simulink model "singletrack_ROS"  (R2017b)
settings: Solver=ode2  StartTime=0.0  StopTime=100  FixedStep=ROS_nodePeriod  MaxStep=1e-3  RelTol=1e-4  AbsTol=1e-4
values from neighbouring files (symbols this model uses):
  initial_conditions = [0,0,0,0,0]    [initParameters.m]
  ROS_clockPublishingPeriod = 1.0e-2    (= 0.01)    [initParameters.m]    (also in init_singletrack.m = 0.0005)
  ROS_nodePeriod = 1.0e-3    (= 0.001)    [initParameters.m]
  ROS_statePublishingPeriod = 2.0e-2    (= 0.02)    [initParameters.m]    (also in init_singletrack.m = 0.01)
undefined symbols (not defined in the file or in its folder): Clock_, Theta, X, Y
libraries: robotlib x12, simulink x1
settings Model: ExtModeTrigDuration=100  Creator=Alessandro  LastModifiedBy=bascetta
settings SolverCC: MaxConsecutiveMinStep=10  ZeroCrossControl=DisableAll
settings DataIOCC: SaveFormat=Array  SaveOutput=off  SaveTime=off  StateSaveName=tmp_raccel_xout  TimeSaveName=t_out  SignalLoggingName=SDO_logsout
settings OptimizationCC: EfficientMapNaN2IntZero=off  LifeSpan=inf
settings DebuggingCC: SFUnexpectedBacktrackingDiag=warning  SFNoUnconditionalDefaultTransitionDiag=warning  SFExecutionAtInitializationDiag=none
settings HardwareCC: ProdBitPerPointer=32  ProdBitPerSizeT=32  ProdBitPerPtrDiffT=32  ProdLargestAtomicFloat=None  ProdIntDivRoundTo=Undefined  ProdEndianess=Unspecified  ProdWordSize=32  ProdHWDeviceType=32-bit Generic  TargetBitPerLong=64  TargetBitPerPointer=64  TargetBitPerSizeT=64  TargetBitPerPtrDiffT=64  TargetLongLongMode=on  TargetIntDivRoundTo=Zero  TargetEndianess=LittleEndian  TargetWordSize=64  TargetHWDeviceType=MATLAB Host  ProdEqTarget=off
settings ModelReferenceCC: PropagateSignalLabelsOutOfModel=off
settings CodeAppCC: MaxIdLength=128  StateflowObjectComments=on
settings GRTTargetCC: TargetLangStandard=C89/C90 (ANSI)  GeneratePreprocessorConditionals=Disable all  CombineOutputUpdateFcns=off  GRTInterface=on
settings ConfigComp: CovMetricSettings=dw  CovHtmlReporting=on  CovSaveCumulativeToWorkspaceVar=on  CovSaveSingleToWorkspaceVar=on  CovExternalEMLEnable=off

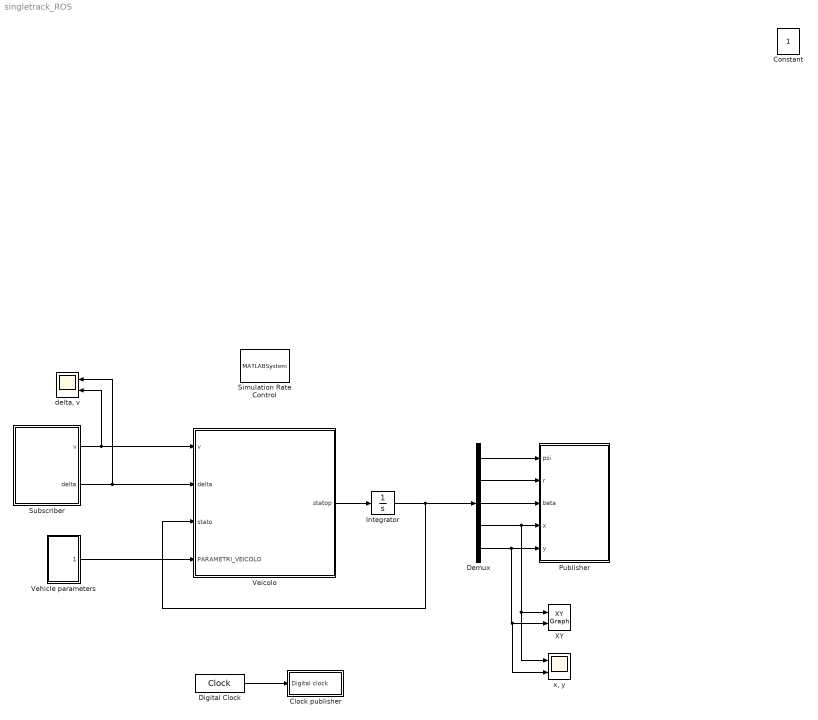
== system singletrack_ROS ==
  Clock publisher : Subsystem
  Demux : Demux  Outputs=5
  Digital Clock : DigitalClock  SampleTime=ROS_nodePeriod
  Integrator : Integrator  InitialCondition=initial_conditions
  Publisher : Subsystem
  Simulation Rate Control : MATLABSystem  System=ExampleHelperSimulationRateControl  SampleTime=ROS_nodePeriod
      mask Type: ExampleHelperSimulationRateControl
      mask Display: disp('Rate Control');
  Subscriber : Subsystem
  Vehicle parameters : Subsystem
  Veicolo : MATLAB Function  TreatAsAtomicUnit=on
  XY : simulink/Sinks/XY Graph  xmin=-5  xmax=5  ymin=-5  ymax=5  st=-1
  "delta, v" : Scope  NumInputPorts=2
  "x, y" : Scope  NumInputPorts=2
  Constant : Constant  IOType=siggen  VectorParams1D=off  SampleTime=1
  wires:
  Digital Clock/1 -> Clock publisher/1(Digital clock)
  Veicolo/1(statop) -> Integrator/1
  Integrator/1 -> Veicolo/3(stato), Demux/1
  Vehicle parameters/1(Params) -> Veicolo/4(PARAMETRI_VEICOLO)
  Subscriber/1(v) -> "delta, v"/2, Veicolo/1(v)
  Subscriber/2(delta) -> "delta, v"/1, Veicolo/2(delta)
  Demux/1 -> Publisher/1(psi)
  Demux/2 -> Publisher/2(r)
  Demux/3 -> Publisher/3(beta)
  Demux/4 -> XY/1, "x, y"/1, Publisher/4(x)
  Demux/5 -> "x, y"/2, XY/2, Publisher/5(y)

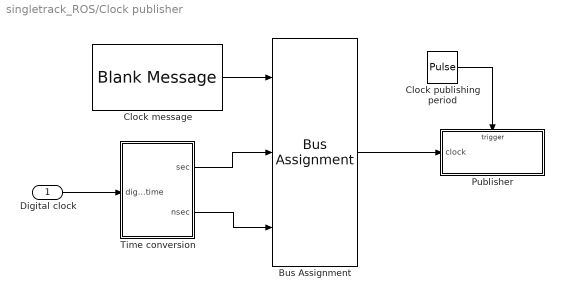
== system singletrack_ROS/Clock publisher ==
  Digital clock : Inport
  Bus Assignment : BusAssignment  DialogController=Simulink.DDGSource_BusAssignment  AssignedSignals=Clock_.Sec,Clock_.Nsec
  Clock message : robotlib/Blank Message  SourceLibraryInfo=This block requires Robotics System Toolbox  messageType=rosgraph_msgs/Clock  SampleTime=inf
      settings: SourceProductBaseCode=RO
  Clock publishing period : DiscretePulseGenerator  PulseType=Time based  Period=ROS_clockPublishingPeriod  PulseWidth=50
  Publisher : Subsystem  TreatAsAtomicUnit=on
  Time conversion : MATLAB Function  TreatAsAtomicUnit=on
  wires:
  Clock message/1 -> Bus Assignment/1
  Bus Assignment/1 -> Publisher/1(clock)
  Time conversion/1(sec) -> Bus Assignment/2
  Time conversion/2(nsec) -> Bus Assignment/3
  Digital clock/1 -> Time conversion/1(digital_time)
  Clock publishing period/1 -> Publisher/Trigger

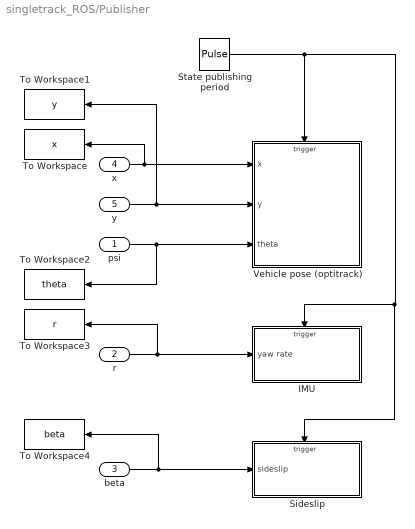
== system singletrack_ROS/Publisher ==
  psi : Inport
  r : Inport  Port=2
  beta : Inport  Port=3
  x : Inport  Port=4
  y : Inport  Port=5
  IMU : Subsystem  TreatAsAtomicUnit=on
  Sideslip : Subsystem  TreatAsAtomicUnit=on
  State publishing period : DiscretePulseGenerator  PulseType=Time based  Period=ROS_statePublishingPeriod  PulseWidth=50
  To Workspace : ToWorkspace  VariableName=x  SampleTime=ROS_nodePeriod
      settings: Save2DSignal=2-D array (concatenate along first dimension)
  To Workspace1 : ToWorkspace  VariableName=y  SampleTime=ROS_nodePeriod
      settings: Save2DSignal=2-D array (concatenate along first dimension)
  To Workspace2 : ToWorkspace  VariableName=theta  SampleTime=ROS_nodePeriod
      settings: Save2DSignal=2-D array (concatenate along first dimension)
  To Workspace3 : ToWorkspace  VariableName=r  SampleTime=ROS_nodePeriod
      settings: Save2DSignal=2-D array (concatenate along first dimension)
  To Workspace4 : ToWorkspace  VariableName=beta  SampleTime=ROS_nodePeriod
      settings: Save2DSignal=2-D array (concatenate along first dimension)
  Vehicle pose (optitrack) : Subsystem  TreatAsAtomicUnit=on
  wires:
  State publishing period/1 -> Sideslip/Trigger, IMU/Trigger, Vehicle pose (optitrack)/Trigger
  x/1 -> To Workspace/1, Vehicle pose (optitrack)/1(x)
  y/1 -> To Workspace1/1, Vehicle pose (optitrack)/2(y)
  psi/1 -> To Workspace2/1, Vehicle pose (optitrack)/3(theta)
  r/1 -> To Workspace3/1, IMU/1(yaw rate)
  beta/1 -> To Workspace4/1, Sideslip/1(sideslip)

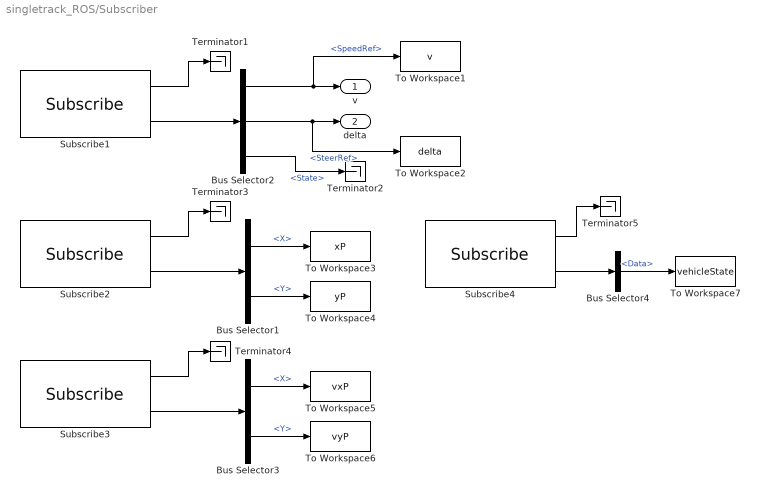
== system singletrack_ROS/Subscriber ==
  Bus Selector1 : BusSelector  OutputSignals=X,Y
  Bus Selector2 : BusSelector  OutputSignals=SpeedRef,SteerRef,State
  Bus Selector3 : BusSelector  OutputSignals=X,Y
  Bus Selector4 : BusSelector  OutputSignals=Data
  Subscribe1 : robotlib/Subscribe  SourceLibraryInfo=This block requires Robotics System Toolbox  topicSource=Specify your own  topic=/controller_cmd  messageType=car_msgs/car_cmd  sampleTime=-1  messageQueueLength=1
      settings: SourceProductBaseCode=RO
  Subscribe2 : robotlib/Subscribe  SourceLibraryInfo=This block requires Robotics System Toolbox  topicSource=Specify your own  topic=/feedback_linearization/pointP  messageType=geometry_msgs/Point  sampleTime=-1  messageQueueLength=1
      settings: SourceProductBaseCode=RO
  Subscribe3 : robotlib/Subscribe  SourceLibraryInfo=This block requires Robotics System Toolbox  topicSource=Specify your own  topic=/feedback_linearization/pointPvelocity  messageType=geometry_msgs/Point  sampleTime=-1  messageQueueLength=1
      settings: SourceProductBaseCode=RO
  Subscribe4 : robotlib/Subscribe  SourceLibraryInfo=This block requires Robotics System Toolbox  topicSource=Specify your own  topic=/feedback_linearization/vehicleState  messageType=std_msgs/Float64MultiArray  sampleTime=-1  messageQueueLength=1
      settings: SourceProductBaseCode=RO
  Terminator{1..5} (5 alike) : Terminator
  To Workspace1 : ToWorkspace  VariableName=v  SampleTime=ROS_nodePeriod
      settings: Save2DSignal=2-D array (concatenate along first dimension)
  To Workspace2 : ToWorkspace  VariableName=delta  SampleTime=ROS_nodePeriod
      settings: Save2DSignal=2-D array (concatenate along first dimension)
  To Workspace3 : ToWorkspace  VariableName=xP  SampleTime=ROS_nodePeriod
      settings: Save2DSignal=2-D array (concatenate along first dimension)
  To Workspace4 : ToWorkspace  VariableName=yP  SampleTime=ROS_nodePeriod
      settings: Save2DSignal=2-D array (concatenate along first dimension)
  To Workspace5 : ToWorkspace  VariableName=vxP  SampleTime=ROS_nodePeriod
      settings: Save2DSignal=2-D array (concatenate along first dimension)
  To Workspace6 : ToWorkspace  VariableName=vyP  SampleTime=ROS_nodePeriod
      settings: Save2DSignal=2-D array (concatenate along first dimension)
  To Workspace7 : ToWorkspace  VariableName=vehicleState  SampleTime=ROS_nodePeriod
      settings: Save2DSignal=2-D array (concatenate along first dimension)
  v : Outport
  delta : Outport  Port=2
  wires:
  Subscribe1/1 -> Terminator1/1
  Subscribe1/2 -> Bus Selector2/1
  Bus Selector2/1 -> To Workspace1/1, v/1  "<SpeedRef>"
  Bus Selector2/2 -> To Workspace2/1, delta/1  "<SteerRef>"
  Bus Selector2/3 -> Terminator2/1  "<State>"
  Subscribe2/1 -> Terminator3/1
  Subscribe2/2 -> Bus Selector1/1
  Bus Selector1/1 -> To Workspace3/1  "<X>"
  Bus Selector1/2 -> To Workspace4/1  "<Y>"
  Bus Selector3/2 -> To Workspace6/1  "<Y>"
  Subscribe3/2 -> Bus Selector3/1
  Subscribe3/1 -> Terminator4/1
  Bus Selector3/1 -> To Workspace5/1  "<X>"
  Subscribe4/1 -> Terminator5/1
  Subscribe4/2 -> Bus Selector4/1
  Bus Selector4/1 -> To Workspace7/1  "<Data>"

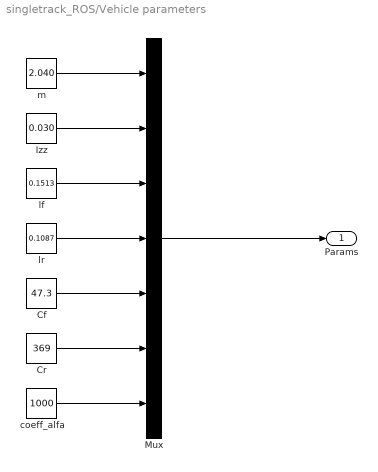
== system singletrack_ROS/Vehicle parameters ==
  Cf : Constant  Value=47.3
  Cr : Constant  Value=369
  Izz : Constant  Value=0.030
  Mux : Mux  Inputs=7
  coeff_alfa : Constant  Value=1000
  lf : Constant  Value=0.1513
  lr : Constant  Value=0.1087
  m : Constant  Value=2.040
  Params : Outport
  wires:
  Mux/1 -> Params/1
  m/1 -> Mux/1
  Izz/1 -> Mux/2
  lf/1 -> Mux/3
  lr/1 -> Mux/4
  Cf/1 -> Mux/5
  Cr/1 -> Mux/6
  coeff_alfa/1 -> Mux/7

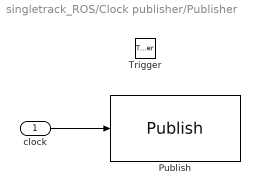
== system singletrack_ROS/Clock publisher/Publisher ==
  clock : Inport
  Trigger : TriggerPort  VariantControl=Variant
  Publish : robotlib/Publish  SourceLibraryInfo=This block requires Robotics System Toolbox  topicSource=Specify your own  topic=/clock  messageType=rosgraph_msgs/Clock  messageQueueLength=1
      settings: SourceProductBaseCode=RO
  wires:
  clock/1 -> Publish/1

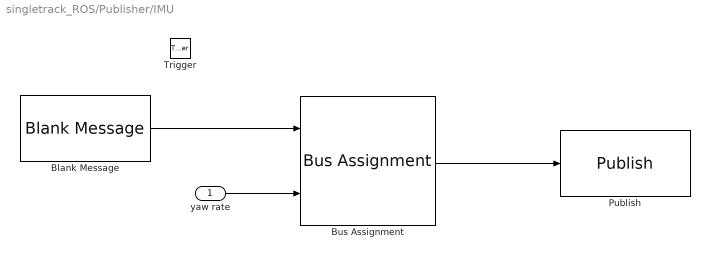
== system singletrack_ROS/Publisher/IMU ==
  yaw rate : Inport
  Trigger : TriggerPort  VariantControl=Variant
  Blank Message : robotlib/Blank Message  SourceLibraryInfo=This block requires Robotics System Toolbox  messageType=sensor_msgs/Imu  SampleTime=inf
      settings: SourceProductBaseCode=RO
  Bus Assignment : BusAssignment  DialogController=Simulink.DDGSource_BusAssignment  AssignedSignals=AngularVelocity.Z
  Publish : robotlib/Publish  SourceLibraryInfo=This block requires Robotics System Toolbox  topicSource=Specify your own  topic=/imu/data  messageType=sensor_msgs/Imu  messageQueueLength=1
      settings: SourceProductBaseCode=RO
  wires:
  Blank Message/1 -> Bus Assignment/1
  Bus Assignment/1 -> Publish/1
  yaw rate/1 -> Bus Assignment/2

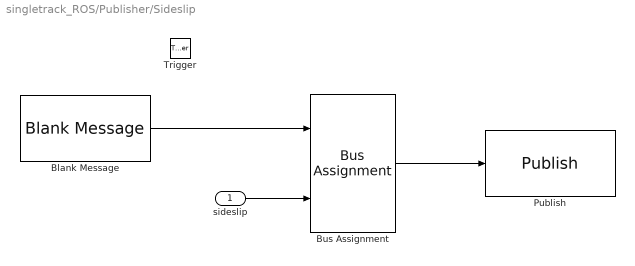
== system singletrack_ROS/Publisher/Sideslip ==
  sideslip : Inport
  Trigger : TriggerPort  VariantControl=Variant
  Blank Message : robotlib/Blank Message  SourceLibraryInfo=This block requires Robotics System Toolbox  messageType=std_msgs/Float64  SampleTime=inf
      settings: SourceProductBaseCode=RO
  Bus Assignment : BusAssignment  DialogController=Simulink.DDGSource_BusAssignment  AssignedSignals=Data
  Publish : robotlib/Publish  SourceLibraryInfo=This block requires Robotics System Toolbox  topicSource=Specify your own  topic=/car_simulator/sideslip  messageType=std_msgs/Float64  messageQueueLength=1
      settings: SourceProductBaseCode=RO
  wires:
  Blank Message/1 -> Bus Assignment/1
  Bus Assignment/1 -> Publish/1
  sideslip/1 -> Bus Assignment/2

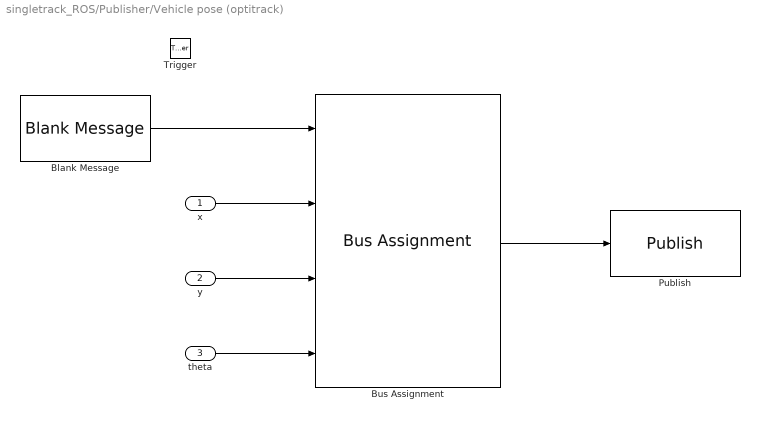
== system singletrack_ROS/Publisher/Vehicle pose (optitrack) ==
  x : Inport
  y : Inport  Port=2
  theta : Inport  Port=3
  Trigger : TriggerPort  VariantControl=Variant
  Blank Message : robotlib/Blank Message  SourceLibraryInfo=This block requires Robotics System Toolbox  messageType=geometry_msgs/Pose2D  SampleTime=inf
      settings: SourceProductBaseCode=RO
  Bus Assignment : BusAssignment  DialogController=Simulink.DDGSource_BusAssignment  AssignedSignals=X,Y,Theta
  Publish : robotlib/Publish  SourceLibraryInfo=This block requires Robotics System Toolbox  topicSource=Specify your own  topic=/car/ground_pose  messageType=geometry_msgs/Pose2D  messageQueueLength=1
      settings: SourceProductBaseCode=RO
  wires:
  Blank Message/1 -> Bus Assignment/1
  Bus Assignment/1 -> Publish/1
  x/1 -> Bus Assignment/2
  y/1 -> Bus Assignment/3
  theta/1 -> Bus Assignment/4

== matlab function singletrack_ROS/Clock publisher/Time conversion ==
  data: digital_time input; sec output; nsec output
function [sec,nsec] = time2rosclock(digital_time)

sec = floor(digital_time);
nsec = round((digital_time-sec)*1.0e+9);

== matlab function singletrack_ROS/Veicolo ==
  data: v input; statop output; delta input; stato input; PARAMETRI_VEICOLO input
function statop =veicolo(v,delta,stato,PARAMETRI_VEICOLO)

m=PARAMETRI_VEICOLO(1);
Izz=PARAMETRI_VEICOLO(2);
lf=PARAMETRI_VEICOLO(3);
lr=PARAMETRI_VEICOLO(4);
Cf=PARAMETRI_VEICOLO(5);
Cr=PARAMETRI_VEICOLO(6);
coeff_alfa=PARAMETRI_VEICOLO(7);

psi=stato(1);
r=stato(2);
beta=stato(3);

if abs(v)>0.1
    psip=r;
    rp=(lr*Cr-lf*Cf)/Izz*beta-(lf^2*Cf+lr^2*Cr)/(v*Izz)*r+lf*Cf/Izz*delta;
    betap=-(Cf+Cr)/(m*v)*beta+(lr*Cr-lf*Cf-m*v^2)/(m*v^2)*r+Cf/(m*v)*delta;
    xp=v*cos(beta+psi);
    yp=v*sin(beta+psi);
else
    psip=0;
    rp=-coeff_alfa*r;
    betap=-coeff_alfa*beta;
    xp=0;
    yp=0;
end

statop=[psip,rp,betap,xp,yp];
